simulink model "task4_dcm"  (R2017a)
settings: Solver=VariableStepAuto  StartTime=0.0  StopTime=0.5  MaxStep=1e-4  RelTol=1e-3
undefined symbols (not defined in the file): Ibase, ki, kis, kp, kps, Vbase
settings Model: Creator=Oskar  LastModifiedBy=Oskar

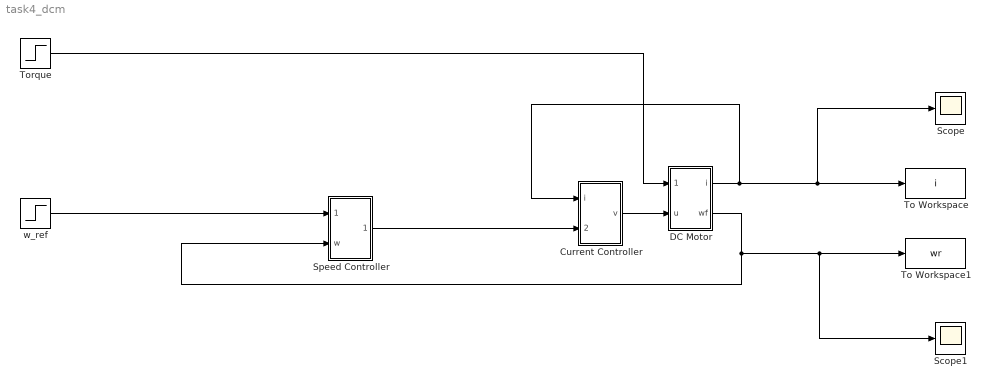
== system task4_dcm ==
  Current Controller : Subsystem
  "DC Motor " : Subsystem  mask{R=0.5, L=2.5/1000, psi=0.35, J=1e-3}
      mask prompts: R "R (ohm)"; L "L (H)"; psi "psi (Vs)"; J "J (kgm^2)"
      mask TypeOptions R: <empty>
  Scope : Scope
  Scope1 : Scope
  Speed Controller : Subsystem
  To Workspace : ToWorkspace  VariableName=i  SaveFormat=Timeseries  SampleTime=-1
  To Workspace1 : ToWorkspace  VariableName=wr  SaveFormat=Timeseries  SampleTime=-1
  Torque : Step  Time=0.1  After=7  SampleTime=0
  "w_ref " : Step  Time=0.3  After=160  SampleTime=0
  wires:
  "DC Motor "/1("i ") -> Current Controller/1(i), Scope/1, To Workspace/1
  "DC Motor "/2("wf ") -> Speed Controller/2(w), Scope1/1, To Workspace1/1
  Torque/1 -> "DC Motor "/1("taul ")
  Current Controller/1(v) -> "DC Motor "/2(u)
  "w_ref "/1 -> Speed Controller/1(w_ref)
  Speed Controller/1(i_ref) -> Current Controller/2("i_ref ")

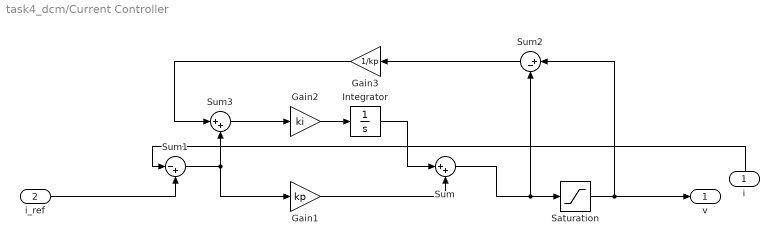
== system task4_dcm/Current Controller ==
  i : Inport
  "i_ref " : Inport  Port=2
  Gain1 : Gain  Gain=kp
  Gain2 : Gain  Gain=ki
  Gain3 : Gain  Gain=1/kp
  Integrator : Integrator
  Saturation : Saturate  UpperLimit=Vbase  LowerLimit=-Vbase
  Sum : Sum  Inputs=|++
  Sum1 : Sum  Inputs=|-+
  Sum2 : Sum  Inputs=|+-
  Sum3 : Sum  Inputs=|++
  v : Outport
  wires:
  "i_ref "/1 -> Sum1/2
  Gain2/1 -> Integrator/1
  Integrator/1 -> Sum/1
  Gain1/1 -> Sum/2
  Saturation/1 -> v/1, Sum2/1
  Sum2/1 -> Gain3/1
  Sum/1 -> Saturation/1, Sum2/2
  Sum1/1 -> Gain1/1, Sum3/2
  Gain3/1 -> Sum3/1
  i/1 -> Sum1/1
  Sum3/1 -> Gain2/1

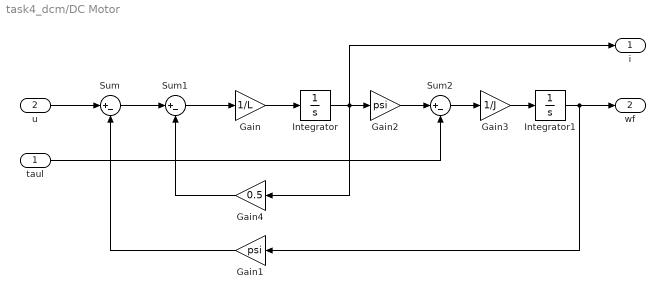
== system task4_dcm/DC Motor  ==
  "taul " : Inport
  u : Inport  Port=2
  Gain : Gain  Gain=1/L
  Gain1 : Gain  Gain=psi
  Gain2 : Gain  Gain=psi
  Gain3 : Gain  Gain=1/J
  Gain4 : Gain  Gain=0.5
  Integrator : Integrator
  Integrator1 : Integrator
  Sum : Sum  Inputs=|+-
  Sum1 : Sum  Inputs=|+-
  Sum2 : Sum  Inputs=|+-
  "i " : Outport
  "wf " : Outport  Port=2
  wires:
  Integrator1/1 -> "wf "/1, Gain1/1
  Sum2/1 -> Gain3/1
  Gain3/1 -> Integrator1/1
  Gain2/1 -> Sum2/1
  Gain4/1 -> Sum1/2
  Sum/1 -> Sum1/1
  u/1 -> Sum/1
  Sum1/1 -> Gain/1
  Gain/1 -> Integrator/1
  "taul "/1 -> Sum2/2
  Integrator/1 -> "i "/1, Gain4/1, Gain2/1
  Gain1/1 -> Sum/2

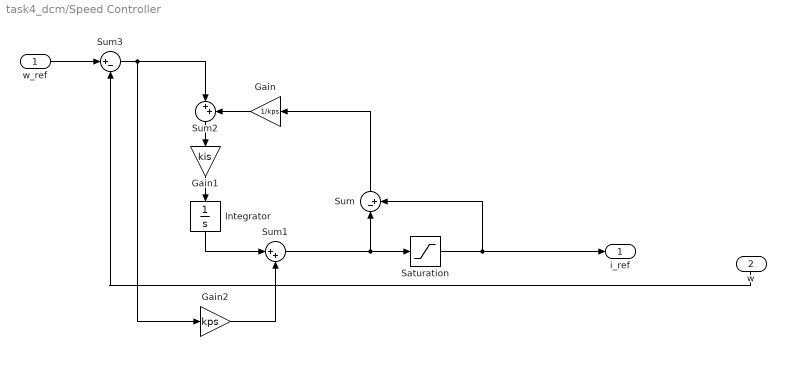
== system task4_dcm/Speed Controller ==
  w_ref : Inport
  w : Inport  Port=2
  Gain : Gain  Gain=1/kps
  Gain1 : Gain  Gain=kis
  Gain2 : Gain  Gain=kps
  Integrator : Integrator
  Saturation : Saturate  UpperLimit=Ibase  LowerLimit=-Ibase
  Sum : Sum  Inputs=|-+
  Sum1 : Sum  Inputs=|++
  Sum2 : Sum  Inputs=|++
  Sum3 : Sum  Inputs=|+-
  i_ref : Outport
  wires:
  Integrator/1 -> Sum1/1
  Gain1/1 -> Integrator/1
  Sum3/1 -> Sum2/1, Gain2/1
  Sum1/1 -> Sum/1, Saturation/1
  w/1 -> Sum3/2
  Gain/1 -> Sum2/2
  Sum2/1 -> Gain1/1
  Sum/1 -> Gain/1
  w_ref/1 -> Sum3/1
  Saturation/1 -> i_ref/1, Sum/2
  Gain2/1 -> Sum1/2
